simulink model "SF043A_TqOscn"  (R2013b)
settings: Solver=FixedStepDiscrete  SolverMode=SingleTasking  StartTime=0.0  StopTime=1  FixedStep=0.002  RelTol=1e-3
values from neighbouring files (symbols this model uses):
  ARCHGLBPRM_2MILLISEC_SEC_F32 = DataDict.Constant    [SF043A_TqOscn_DataDict.m]
  ARCHGLBPRM_2PI_ULS_F32 = DataDict.Constant    [SF043A_TqOscn_DataDict.m]
  DCTHD_MOTNWTMTR_F32 = DataDict.Constant    [SF043A_TqOscn_DataDict.m]
  DFTFALLRAMPRATE_MOTNWTMTRPERSEC_F32 = DataDict.Constant    [SF043A_TqOscn_DataDict.m]
  DFTPHAAGINC_MATRAD_F32 = DataDict.Constant    [SF043A_TqOscn_DataDict.m]
  DFTRISNGRAMPRATE_MOTNWTMTRPERSEC_F32 = DataDict.Constant    [SF043A_TqOscn_DataDict.m]
  FltInj_f32 = DataDict.Client    [SF043A_TqOscn_DataDict.m]
  FLTINJ_TQOSCN_PREFINALCMD = DataDict.Constant    [SF043A_TqOscn_DataDict.m]
  MAXAMP_MOTNWTMTR_F32 = DataDict.Constant    [SF043A_TqOscn_DataDict.m]
  MAXRAMPRATE_MOTNWTMTR_F32 = DataDict.Constant    [SF043A_TqOscn_DataDict.m]
  MINAMP_MOTNWTMTR_F32 = DataDict.Constant    [SF043A_TqOscn_DataDict.m]
  MINRAMPRATE_MOTNWTMTR_F32 = DataDict.Constant    [SF043A_TqOscn_DataDict.m]
  TqOscnAmpLimY = DataDict.Calibration    [SF043A_TqOscn_DataDict.m]
  TqOscnFallRampRateCal = DataDict.Calibration    [SF043A_TqOscn_DataDict.m]
  TqOscnFrqIn = DataDict.Calibration    [SF043A_TqOscn_DataDict.m]
  TqOscnRisngRampRateCal = DataDict.Calibration    [SF043A_TqOscn_DataDict.m]
  TqOscnUseRampRateCal = DataDict.Calibration    [SF043A_TqOscn_DataDict.m]
libraries: NxtrLim x6, simulink x3, NxtrAbslt x3, Fil x2, FixdToFloat x2, autosarlib x1, NxtrMath x1, FloatToFixd x1
(part 2 of 2)

== system SF043A_TqOscn/TqOscn/TqOscnPer1/DC Check/DC_ok ==
  In1 : Inport
  Action Port : ActionPort  ActionType=else
  Constant1 : Constant  Value=false  OutDataTypeStr=boolean
      settings: AttributesFormatString=%<OutDataTypeStr>
  CopyRight2 : Subsystem  Description=|  mask(Copyright Information){none=on}
      | Copyright info block.                                               
      |                                                                     
      | Place copyright information at the top of every subsystem in design.
      mask prompts: none "No parameters"
      mask help: Place copyright information at the top of every subsystem in design.
      mask Display:
      | NxtrConf = 'Nexteer Confidential';
      | 
      | sys = bdroot; %handle for the current model ("system")
      | first = get_param(sys,'Created');
      | if(isempty(first))
      |     first = datestr(now,'yyyy');
      | else
      |     first = first(end-3:end);  %year is last four digits
      | end
      | 
      | last = get_param(sys,'LastModifiedDate');
      | if isempty(last)
      |     last = datestr(now,'yyyy');
      | else
      |     last = last(end-3:end);
      | end
      | 
      | if strcmp(first,last)
      |     fprintf('%s -- Copyright %s Nexteer',NxtrConf,first)
      | else
      |     fprintf('%s -- %s%s- %s Nexteer',NxtrConf,char(169),first,last)
      | end
  Cmd : Outport
  Excdd : Outport  Port=2
  wires:
  In1/1 -> Cmd/1
  Constant1/1 -> Excdd/1

== system SF043A_TqOscn/TqOscn/TqOscnPer1/FltInj_f32 client/CodeGen ==
  note: NOTE 1:  Simulink 2013b cannot handle InOut arguments, so the operation
      |                 prototype inside this block is not quite right.
      |
      | NOTE 2:  Do not use this variant for simulation.  Sig_Out = zero, always.
  note: FltInj_f32(float32 *SigPah, uint16 LocnKey)
  Sig : Inport
  "LocnKey  " : Inport  Port=2
  CopyRight1 : Subsystem  Description=|  mask(Copyright Information){none=on}
      | Copyright info block.                                               
      |                                                                     
      | Place copyright information at the top of every subsystem in design.
      mask prompts: none "No parameters"
      mask help: Place copyright information at the top of every subsystem in design.
      mask Display:
      | NxtrConf = 'Nexteer Confidential';
      | 
      | sys = bdroot; %handle for the current model ("system")
      | first = get_param(sys,'Created');
      | if(isempty(first))
      |     first = datestr(now,'yyyy');
      | else
      |     first = first(end-3:end);  %year is last four digits
      | end
      | 
      | last = get_param(sys,'LastModifiedDate');
      | if isempty(last)
      |     last = datestr(now,'yyyy');
      | else
      |     last = last(end-3:end);
      | end
      | 
      | if strcmp(first,last)
      |     fprintf('%s -- Copyright %s Nexteer',NxtrConf,first)
      | else
      |     fprintf('%s -- %s%s- %s Nexteer',NxtrConf,char(169),first,last)
      | end
  Invoke AUTOSAR Server Operation : autosarlib/Invoke AUTOSAR Server Operation  portName=FltInj_f32  operationPrototype=FltInj_f32(IN single SigPah_ArgIn, OUT single SigPah_ArgOut, IN uint16 LocnKey)  interfacePath=/AUTOSAR/Interface  serverType=Application software  showErrorStatus=off  SAMPLETIME=-1  showARPortLabels=on
  Sig_Out : Outport  OutDataTypeStr=single
  wires:
  Sig/1 -> Invoke AUTOSAR Server Operation/1
  "LocnKey  "/1 -> Invoke AUTOSAR Server Operation/2
  Invoke AUTOSAR Server Operation/1 -> Sig_Out/1

== system SF043A_TqOscn/TqOscn/TqOscnPer1/FltInj_f32 client/CopyRight1 ==

== system SF043A_TqOscn/TqOscn/TqOscnPer1/FltInj_f32 client/Sim ==
  note: This block requires no modification by FDD author.
      |
      | This block does not actually simulate any fault injection.  It is simply a pass-thru.
      |
      | Input port (#2) simply terminates its signal, but we are trying to force the FDD author
      | to properly use the FltInjectionLocType enumeration in FDD model.
  note: EA4.x Fault Injection
  Sig : Inport
  "LocnKey  " : Inport  Port=2  OutDataTypeStr=uint16
  CopyRight1 : Subsystem  Description=|  mask(Copyright Information){none=on}
      | Copyright info block.                                               
      |                                                                     
      | Place copyright information at the top of every subsystem in design.
      mask prompts: none "No parameters"
      mask help: Place copyright information at the top of every subsystem in design.
      mask Display:
      | NxtrConf = 'Nexteer Confidential';
      | 
      | sys = bdroot; %handle for the current model ("system")
      | first = get_param(sys,'Created');
      | if(isempty(first))
      |     first = datestr(now,'yyyy');
      | else
      |     first = first(end-3:end);  %year is last four digits
      | end
      | 
      | last = get_param(sys,'LastModifiedDate');
      | if isempty(last)
      |     last = datestr(now,'yyyy');
      | else
      |     last = last(end-3:end);
      | end
      | 
      | if strcmp(first,last)
      |     fprintf('%s -- Copyright %s Nexteer',NxtrConf,first)
      | else
      |     fprintf('%s -- %s%s- %s Nexteer',NxtrConf,char(169),first,last)
      | end
  Terminator : Terminator
  Sig_Out : Outport
  wires:
  Sig/1 -> Sig_Out/1
  "LocnKey  "/1 -> Terminator/1

== system SF043A_TqOscn/TqOscn/TqOscnPer1/Set_false/CopyRight2 ==

== system SF043A_TqOscn/TqOscn/TqOscnPer1/Set_true/CopyRight2 ==

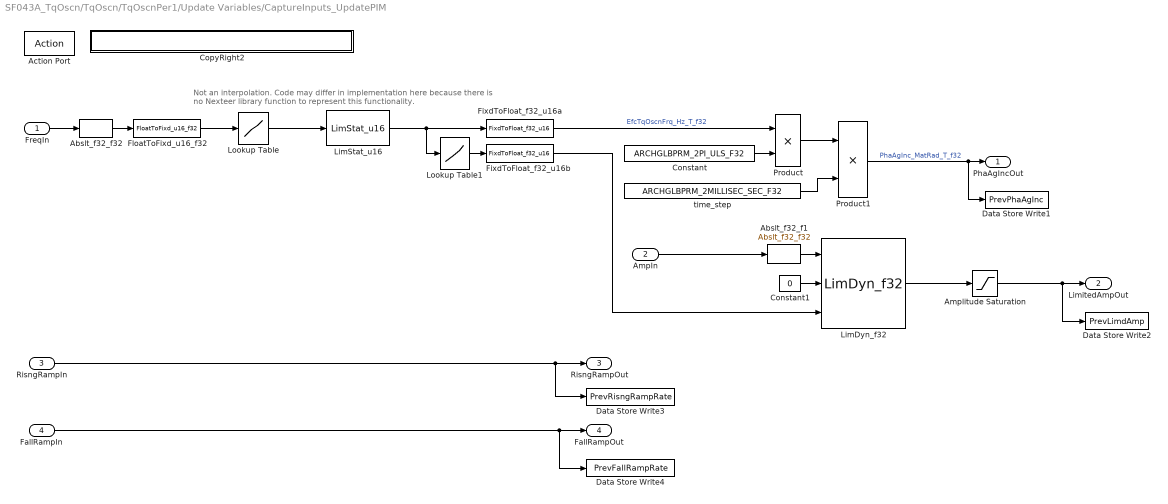
== system SF043A_TqOscn/TqOscn/TqOscnPer1/Update Variables/CaptureInputs_UpdatePIM ==
  note: Not an interpolation.  Code may differ in implementation here because there
      | is no Nexteer library function to represent this functionality.
  FreqIn : Inport
  AmpIn : Inport  Port=2
  RisngRampIn : Inport  Port=3
  FallRampIn : Inport  Port=4
  Action Port : ActionPort  ActionType=then
  Abslt_f32_f1 : NxtrAbslt/Abslt_f32_f32  SFunctionSpec=single y1 = Abslt_f32_f32(single u1)
      settings: AttributesFormatString=%<Name>
  Abslt_f32_f32 : NxtrAbslt/Abslt_f32_f32  SFunctionSpec=single y1 = Abslt_f32_f32(single u1)
      settings: AttributesFormatString=%<Name>
  Amplitude Saturation : Saturate  UpperLimit=MAXAMP_MOTNWTMTR_F32  LowerLimit=MINAMP_MOTNWTMTR_F32
      settings: AttributesFormatString=UPR=%<UpperLimit>\nLWR=%<LowerLimit>
  Constant : Constant  Value=ARCHGLBPRM_2PI_ULS_F32
  Constant1 : Constant  Value=0  OutDataTypeStr=single
      settings: AttributesFormatString=%<OutDataTypeStr>
  CopyRight2 : Subsystem  Description=|  mask(Copyright Information){none=on}
      | Copyright info block.                                               
      |                                                                     
      | Place copyright information at the top of every subsystem in design.
      mask prompts: none "No parameters"
      mask help: Place copyright information at the top of every subsystem in design.
      mask Display:
      | NxtrConf = 'Nexteer Confidential';
      | 
      | sys = bdroot; %handle for the current model ("system")
      | first = get_param(sys,'Created');
      | if(isempty(first))
      |     first = datestr(now,'yyyy');
      | else
      |     first = first(end-3:end);  %year is last four digits
      | end
      | 
      | last = get_param(sys,'LastModifiedDate');
      | if isempty(last)
      |     last = datestr(now,'yyyy');
      | else
      |     last = last(end-3:end);
      | end
      | 
      | if strcmp(first,last)
      |     fprintf('%s -- Copyright %s Nexteer',NxtrConf,first)
      | else
      |     fprintf('%s -- %s%s- %s Nexteer',NxtrConf,char(169),first,last)
      | end
  Data Store Write1 : DataStoreWrite  DataStoreName=PrevPhaAgInc
  Data Store Write2 : DataStoreWrite  DataStoreName=PrevLimdAmp
  Data Store Write3 : DataStoreWrite  DataStoreName=PrevRisngRampRate
  Data Store Write4 : DataStoreWrite  DataStoreName=PrevFallRampRate
  FixdToFloat_f32_u16a : FixdToFloat/FixdToFloat_f32_u16  Param1=8
  FixdToFloat_f32_u16b : FixdToFloat/FixdToFloat_f32_u16  Param1=11
  FloatToFixd_u16_f32 : FloatToFixd/FloatToFixd_u16_f32  Param1=8
  LimDyn_f32 : NxtrLim/LimDyn_f32
  LimStat_u16 : NxtrLim/LimStat_u16  LoLim=MINFRQ_CNT_U16  HiLim=MAXFRQ_CNT_U16
      settings: AttributesFormatString=|
      | Low Limit: %<LoLim>
      | High Limit:%<HiLim>
  Lookup Table : Lookup  InputValues=TqOscnFrqIn  Table=TqOscnFrqIn  LookUpMeth=Use Input Below
      settings: AttributesFormatString=Input=%<InputValues>\nOutput=%<OutputValues>\nLookup Method=\n%<LookUpMeth>
  Lookup Table1 : Lookup  InputValues=TqOscnFrqIn  Table=TqOscnAmpLimY  LookUpMeth=Use Input Below
      settings: AttributesFormatString=Input=%<InputValues>\nOutput=%<OutputValues>\nLookup Method=\n%<LookUpMeth>
  Product : Product  RndMeth=Zero
  Product1 : Product  RndMeth=Zero
  time_step : Constant  Value=ARCHGLBPRM_2MILLISEC_SEC_F32
  PhaAgIncOut : Outport
  LimitedAmpOut : Outport  Port=2
  RisngRampOut : Outport  Port=3
  FallRampOut : Outport  Port=4
  wires:
  AmpIn/1 -> Abslt_f32_f1/1
  Lookup Table/1 -> LimStat_u16/1
  LimStat_u16/1 -> FixdToFloat_f32_u16a/1, Lookup Table1/1
  Product/1 -> Product1/1
  time_step/1 -> Product1/2
  LimDyn_f32/1 -> Amplitude Saturation/1
  FreqIn/1 -> Abslt_f32_f32/1
  Lookup Table1/1 -> FixdToFloat_f32_u16b/1
  Constant/1 -> Product/2
  Abslt_f32_f1/1 -> LimDyn_f32/1
  Abslt_f32_f32/1 -> FloatToFixd_u16_f32/1
  Amplitude Saturation/1 -> Data Store Write2/1, LimitedAmpOut/1
  Product1/1 -> Data Store Write1/1, PhaAgIncOut/1  "PhaAgInc_MatRad_T_f32"
  FallRampIn/1 -> Data Store Write4/1, FallRampOut/1
  Constant1/1 -> LimDyn_f32/2
  RisngRampIn/1 -> Data Store Write3/1, RisngRampOut/1
  FloatToFixd_u16_f32/1 -> Lookup Table/1
  FixdToFloat_f32_u16a/1 -> Product/1  "EfcTqOscnFrq_Hz_T_f32"
  FixdToFloat_f32_u16b/1 -> LimDyn_f32/3

== system SF043A_TqOscn/TqOscn/TqOscnPer1/Update Variables/CopyRight2 ==

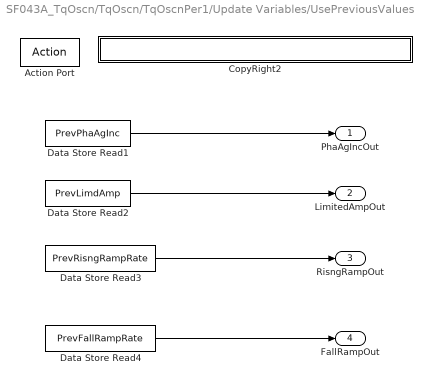
== system SF043A_TqOscn/TqOscn/TqOscnPer1/Update Variables/UsePreviousValues ==
  Action Port : ActionPort  ActionType=else
  CopyRight2 : Subsystem  Description=|  mask(Copyright Information){none=on}
      | Copyright info block.                                               
      |                                                                     
      | Place copyright information at the top of every subsystem in design.
      mask prompts: none "No parameters"
      mask help: Place copyright information at the top of every subsystem in design.
      mask Display:
      | NxtrConf = 'Nexteer Confidential';
      | 
      | sys = bdroot; %handle for the current model ("system")
      | first = get_param(sys,'Created');
      | if(isempty(first))
      |     first = datestr(now,'yyyy');
      | else
      |     first = first(end-3:end);  %year is last four digits
      | end
      | 
      | last = get_param(sys,'LastModifiedDate');
      | if isempty(last)
      |     last = datestr(now,'yyyy');
      | else
      |     last = last(end-3:end);
      | end
      | 
      | if strcmp(first,last)
      |     fprintf('%s -- Copyright %s Nexteer',NxtrConf,first)
      | else
      |     fprintf('%s -- %s%s- %s Nexteer',NxtrConf,char(169),first,last)
      | end
  Data Store Read1 : DataStoreRead  DataStoreName=PrevPhaAgInc
  Data Store Read2 : DataStoreRead  DataStoreName=PrevLimdAmp
  Data Store Read3 : DataStoreRead  DataStoreName=PrevRisngRampRate
  Data Store Read4 : DataStoreRead  DataStoreName=PrevFallRampRate
  PhaAgIncOut : Outport
  LimitedAmpOut : Outport  Port=2
  RisngRampOut : Outport  Port=3
  FallRampOut : Outport  Port=4
  wires:
  Data Store Read4/1 -> FallRampOut/1
  Data Store Read3/1 -> RisngRampOut/1
  Data Store Read1/1 -> PhaAgIncOut/1
  Data Store Read2/1 -> LimitedAmpOut/1

== system SF043A_TqOscn/TqOscn/TqOscnPer1/Amplitude Rate Limiter/SetToZero/CopyRight2 ==

== system SF043A_TqOscn/TqOscn/TqOscnPer1/Amplitude Rate Limiter/UseCals/CopyRight2 ==

== system SF043A_TqOscn/TqOscn/TqOscnPer1/Angle Wrapper/Pass_through/CopyRight2 ==

== system SF043A_TqOscn/TqOscn/TqOscnPer1/Angle Wrapper/Subtract_2pi/CopyRight2 ==

== system SF043A_TqOscn/TqOscn/TqOscnPer1/CheckFlag/SetToZero/CopyRight2 ==

== system SF043A_TqOscn/TqOscn/TqOscnPer1/CheckFlag/UseInput/CopyRight2 ==

== system SF043A_TqOscn/TqOscn/TqOscnPer1/DC Check/DC Trend/CopyRight2 ==

== system SF043A_TqOscn/TqOscn/TqOscnPer1/DC Check/DC_Detd/CopyRight2 ==

== system SF043A_TqOscn/TqOscn/TqOscnPer1/DC Check/DC_ok/CopyRight2 ==

== system SF043A_TqOscn/TqOscn/TqOscnPer1/FltInj_f32 client/CodeGen/CopyRight1 ==

== system SF043A_TqOscn/TqOscn/TqOscnPer1/FltInj_f32 client/Sim/CopyRight1 ==

== system SF043A_TqOscn/TqOscn/TqOscnPer1/Update Variables/CaptureInputs_UpdatePIM/CopyRight2 ==

== system SF043A_TqOscn/TqOscn/TqOscnPer1/Update Variables/UsePreviousValues/CopyRight2 ==
